simulink model "SWC_DDM_type"  (R2021b)
settings: Solver=FixedStepDiscrete  StartTime=0.0  StopTime=10.0  FixedStep=0.01  RelTol=1e-3
undefined symbols (not defined in the file): C_TASK_5MS_S, FALSE, TRUE
libraries: ddm x1
settings Model: DataDictionary=APPTypes.sldd  Creator=FVT23010  LastModifiedBy=FVT23010
settings DataIOCC: SaveFormat=StructureWithTime
settings OptimizationCC: DefaultParameterBehavior=Inlined  EnhancedBackFolding=on  PassReuseOutputArgsAs=Individual arguments  ZeroExternalMemoryAtStartup=off  ZeroInternalMemoryAtStartup=off  OptimizeBlockOrder=speed  DifferentSizesBufferReuse=on  OptimizationCustomize=off  EfficientTunableParamExpr=on
settings DebuggingCC: ParameterTunabilityLossMsg=error
settings HardwareCC: ProdBitPerPointer=32  ProdBitPerSizeT=32  ProdBitPerPtrDiffT=32  ProdLargestAtomicInteger=Long  ProdLargestAtomicFloat=Double  ProdWordSize=32  ProdLongLongMode=on  ProdHWDeviceType=ARM Compatible->ARM Cortex-M
settings ModelReferenceCC: ModelReferenceNumInstancesAllowed=Single
settings SFSimCC: MATLABDynamicMemAlloc=off
settings RTWCC: Description=AUTOSAR  SystemTargetFile=autosar.tlc  GenCodeOnly=on  TemplateMakefile=ert_default_tmf  PortableWordSizes=on
settings CodeAppCC: ForceParamTrailComments=on  IgnoreCustomStorageClasses=off  OperatorAnnotations=on  SimulinkDataObjDesc=on  SFDataObjDesc=on  InsertBlockDesc=on
settings STFCustomTargetCC: TargetLangStandard=C99 (ISO)  UtilityFuncGeneration=Shared location  MultiwordLength=256  ParMdlRefBuildCompliant=on  CompOptLevelCompliant=on  IncludeMdlTerminateFcn=off  CombineOutputUpdateFcns=on  SuppressErrorStatus=on  ERTCustomFileBanners=on  SupportNonFinite=off  SupportComplex=off  SupportContinuousTime=off  SupportNonInlinedSFcns=off  RemoveResetFunc=on  MATLABClassNameForMDSCustomization=Simulink.SoftwareTarget.ERTCustomization  AutosarCompliant=on  GRTInterface=off  UseToolchainInfoCompliant=on  GenerateSharedConstants=off  LookupTableObjectStructAxisOrder=2,1,3,4,...  LUTObjectStructOrderEvenSpacing=Size,Table,Breakpoints  SystemTargetFile=autosar.tlc
settings ERTTargetCC: TargetLangStandard=C99 (ISO)  UtilityFuncGeneration=Shared location  ConcurrentExecutionCompliant=off  IncludeMdlTerminateFcn=off  SuppressErrorStatus=on  SupportNonFinite=off  SupportComplex=off  ModelStepFunctionPrototypeControlCompliant=off  CPPClassGenCompliant=off  AutosarCompliant=on  GenerateSharedConstants=off  LookupTableObjectStructAxisOrder=2,1,3,4,...  LUTObjectStructOrderEvenSpacing=Size,Table,Breakpoints  GenerateASAP2=on  InlinedParameterPlacement=NonHierarchical  ERTCustomFileTemplate=example_file_process.tlc  ConvertIfToSwitch=off  SuppressUnreachableDefaultCases=off  BooleanTrueId=true_MatlabRTW  BooleanFalseId=false_MatlabRTW

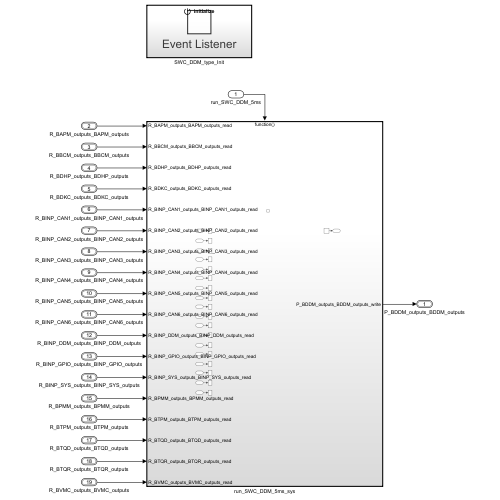
[thumbnail: Simulink's stored preview of the top-level diagram]
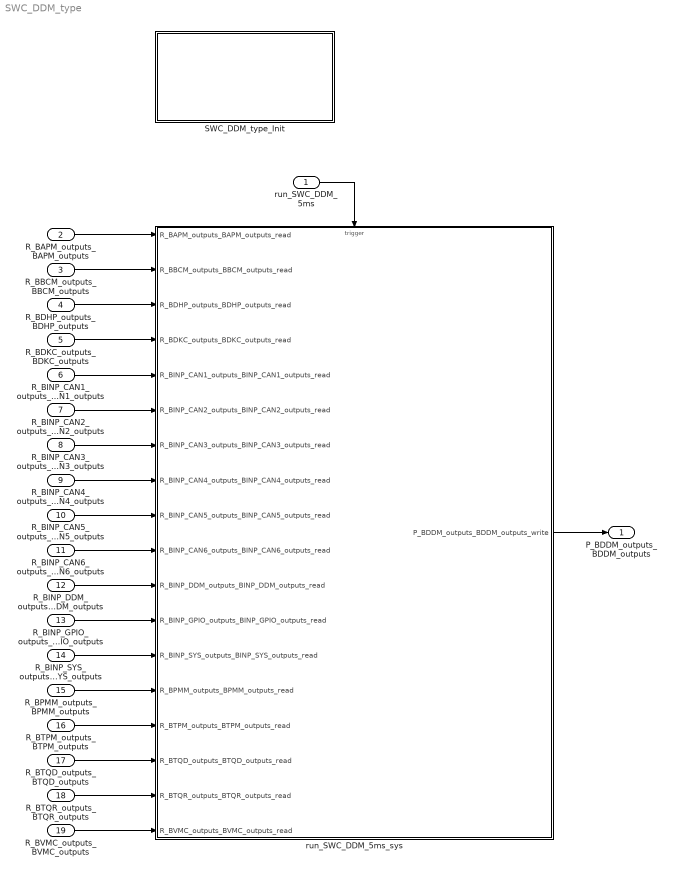
== system SWC_DDM_type ==
  run_SWC_DDM_5ms : Inport  SampleTime=0.01  OutputFunctionCall=on
  R_BAPM_outputs_BAPM_outputs : Inport  Port=2  OutDataTypeStr=Bus: BAPM_outputs  PortDimensions=1  BusOutputAsStruct=on
  R_BBCM_outputs_BBCM_outputs : Inport  Port=3  OutDataTypeStr=Bus: BBCM_outputs  PortDimensions=1  BusOutputAsStruct=on
  R_BDHP_outputs_BDHP_outputs : Inport  Port=4  OutDataTypeStr=Bus: BDHP_outputs  PortDimensions=1  BusOutputAsStruct=on
  R_BDKC_outputs_BDKC_outputs : Inport  Port=5  OutDataTypeStr=Bus: BDKC_outputs  PortDimensions=1  BusOutputAsStruct=on
  R_BINP_CAN1_outputs_BINP_CAN1_outputs : Inport  Port=6  OutDataTypeStr=Bus: BINP_CAN1_outputs  PortDimensions=1  BusOutputAsStruct=on
  R_BINP_CAN2_outputs_BINP_CAN2_outputs : Inport  Port=7  OutDataTypeStr=Bus: BINP_CAN2_outputs  PortDimensions=1  BusOutputAsStruct=on
  R_BINP_CAN3_outputs_BINP_CAN3_outputs : Inport  Port=8  OutDataTypeStr=Bus: BINP_CAN3_outputs  PortDimensions=1  BusOutputAsStruct=on
  R_BINP_CAN4_outputs_BINP_CAN4_outputs : Inport  Port=9  OutDataTypeStr=Bus: BINP_CAN4_outputs  PortDimensions=1  BusOutputAsStruct=on
  R_BINP_CAN5_outputs_BINP_CAN5_outputs : Inport  Port=10  OutDataTypeStr=Bus: BINP_CAN5_outputs  PortDimensions=1  BusOutputAsStruct=on
  R_BINP_CAN6_outputs_BINP_CAN6_outputs : Inport  Port=11  OutDataTypeStr=Bus: BINP_CAN6_outputs  PortDimensions=1  BusOutputAsStruct=on
  R_BINP_DDM_outputs_BINP_DDM_outputs : Inport  Port=12  OutDataTypeStr=Bus: BINP_DDM_outputs  PortDimensions=1  BusOutputAsStruct=on
  R_BINP_GPIO_outputs_BINP_GPIO_outputs : Inport  Port=13  OutDataTypeStr=Bus: BINP_GPIO_outputs  PortDimensions=1  BusOutputAsStruct=on
  R_BINP_SYS_outputs_BINP_SYS_outputs : Inport  Port=14  OutDataTypeStr=Bus: BINP_SYS_outputs  PortDimensions=1  BusOutputAsStruct=on
  R_BPMM_outputs_BPMM_outputs : Inport  Port=15  OutDataTypeStr=Bus: BPMM_outputs  PortDimensions=1  BusOutputAsStruct=on
  R_BTPM_outputs_BTPM_outputs : Inport  Port=16  OutDataTypeStr=Bus: BTPM_outputs  PortDimensions=1  BusOutputAsStruct=on
  R_BTQD_outputs_BTQD_outputs : Inport  Port=17  OutDataTypeStr=Bus: BTQD_outputs  PortDimensions=1  BusOutputAsStruct=on
  R_BTQR_outputs_BTQR_outputs : Inport  Port=18  OutDataTypeStr=Bus: BTQR_outputs  PortDimensions=1  BusOutputAsStruct=on
  R_BVMC_outputs_BVMC_outputs : Inport  Port=19  OutDataTypeStr=Bus: BVMC_outputs  PortDimensions=1  BusOutputAsStruct=on
  SWC_DDM_type_Init : Subsystem
  run_SWC_DDM_5ms_sys : Subsystem
  P_BDDM_outputs_BDDM_outputs : Outport  OutDataTypeStr=Bus: BDDM_outputs  PortDimensions=1  BusOutputAsStruct=on
  wires:
  R_BAPM_outputs_BAPM_outputs/1 -> run_SWC_DDM_5ms_sys/1(R_BAPM_outputs_BAPM_outputs_read)
  R_BBCM_outputs_BBCM_outputs/1 -> run_SWC_DDM_5ms_sys/2(R_BBCM_outputs_BBCM_outputs_read)
  R_BDHP_outputs_BDHP_outputs/1 -> run_SWC_DDM_5ms_sys/3(R_BDHP_outputs_BDHP_outputs_read)
  R_BDKC_outputs_BDKC_outputs/1 -> run_SWC_DDM_5ms_sys/4(R_BDKC_outputs_BDKC_outputs_read)
  R_BINP_CAN1_outputs_BINP_CAN1_outputs/1 -> run_SWC_DDM_5ms_sys/5(R_BINP_CAN1_outputs_BINP_CAN1_outputs_read)
  R_BINP_CAN2_outputs_BINP_CAN2_outputs/1 -> run_SWC_DDM_5ms_sys/6(R_BINP_CAN2_outputs_BINP_CAN2_outputs_read)
  R_BINP_CAN3_outputs_BINP_CAN3_outputs/1 -> run_SWC_DDM_5ms_sys/7(R_BINP_CAN3_outputs_BINP_CAN3_outputs_read)
  R_BINP_CAN4_outputs_BINP_CAN4_outputs/1 -> run_SWC_DDM_5ms_sys/8(R_BINP_CAN4_outputs_BINP_CAN4_outputs_read)
  R_BINP_CAN5_outputs_BINP_CAN5_outputs/1 -> run_SWC_DDM_5ms_sys/9(R_BINP_CAN5_outputs_BINP_CAN5_outputs_read)
  R_BINP_CAN6_outputs_BINP_CAN6_outputs/1 -> run_SWC_DDM_5ms_sys/10(R_BINP_CAN6_outputs_BINP_CAN6_outputs_read)
  R_BINP_DDM_outputs_BINP_DDM_outputs/1 -> run_SWC_DDM_5ms_sys/11(R_BINP_DDM_outputs_BINP_DDM_outputs_read)
  R_BINP_GPIO_outputs_BINP_GPIO_outputs/1 -> run_SWC_DDM_5ms_sys/12(R_BINP_GPIO_outputs_BINP_GPIO_outputs_read)
  R_BINP_SYS_outputs_BINP_SYS_outputs/1 -> run_SWC_DDM_5ms_sys/13(R_BINP_SYS_outputs_BINP_SYS_outputs_read)
  R_BPMM_outputs_BPMM_outputs/1 -> run_SWC_DDM_5ms_sys/14(R_BPMM_outputs_BPMM_outputs_read)
  R_BTPM_outputs_BTPM_outputs/1 -> run_SWC_DDM_5ms_sys/15(R_BTPM_outputs_BTPM_outputs_read)
  R_BTQD_outputs_BTQD_outputs/1 -> run_SWC_DDM_5ms_sys/16(R_BTQD_outputs_BTQD_outputs_read)
  R_BTQR_outputs_BTQR_outputs/1 -> run_SWC_DDM_5ms_sys/17(R_BTQR_outputs_BTQR_outputs_read)
  R_BVMC_outputs_BVMC_outputs/1 -> run_SWC_DDM_5ms_sys/18(R_BVMC_outputs_BVMC_outputs_read)
  run_SWC_DDM_5ms_sys/1(P_BDDM_outputs_BDDM_outputs_write) -> P_BDDM_outputs_BDDM_outputs/1
  run_SWC_DDM_5ms/1 -> run_SWC_DDM_5ms_sys/Trigger

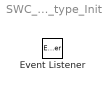
== system SWC_DDM_type/SWC_DDM_type_Init ==
  Event Listener : EventListener  EventName=reset

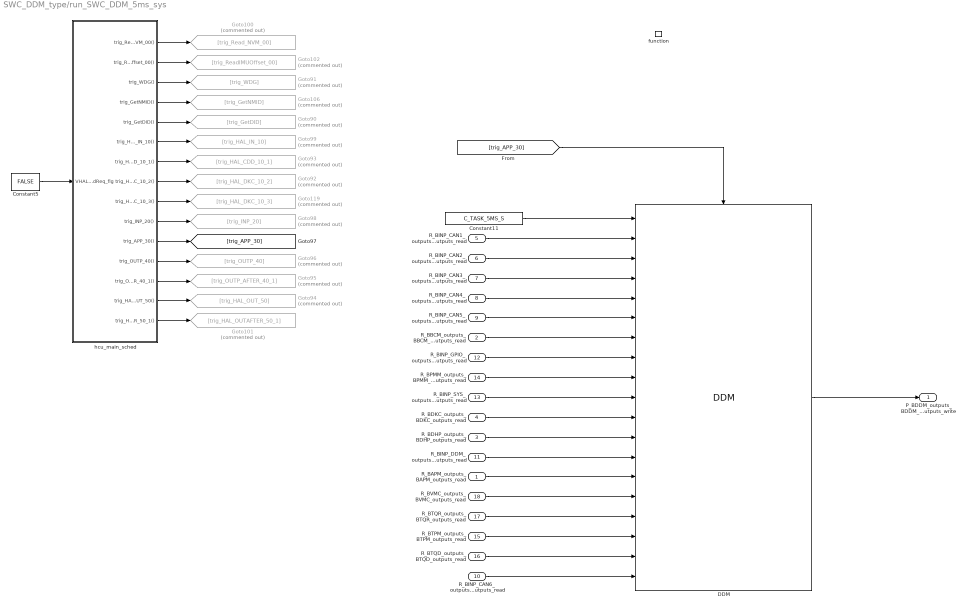
== system SWC_DDM_type/run_SWC_DDM_5ms_sys ==
  R_BAPM_outputs_BAPM_outputs_read : Inport
  R_BBCM_outputs_BBCM_outputs_read : Inport  Port=2
  R_BDHP_outputs_BDHP_outputs_read : Inport  Port=3
  R_BDKC_outputs_BDKC_outputs_read : Inport  Port=4
  R_BINP_CAN1_outputs_BINP_CAN1_outputs_read : Inport  Port=5
  R_BINP_CAN2_outputs_BINP_CAN2_outputs_read : Inport  Port=6
  R_BINP_CAN3_outputs_BINP_CAN3_outputs_read : Inport  Port=7
  R_BINP_CAN4_outputs_BINP_CAN4_outputs_read : Inport  Port=8
  R_BINP_CAN5_outputs_BINP_CAN5_outputs_read : Inport  Port=9
  R_BINP_CAN6_outputs_BINP_CAN6_outputs_read : Inport  Port=10
  R_BINP_DDM_outputs_BINP_DDM_outputs_read : Inport  Port=11
  R_BINP_GPIO_outputs_BINP_GPIO_outputs_read : Inport  Port=12
  R_BINP_SYS_outputs_BINP_SYS_outputs_read : Inport  Port=13
  R_BPMM_outputs_BPMM_outputs_read : Inport  Port=14
  R_BTPM_outputs_BTPM_outputs_read : Inport  Port=15
  R_BTQD_outputs_BTQD_outputs_read : Inport  Port=16
  R_BTQR_outputs_BTQR_outputs_read : Inport  Port=17
  R_BVMC_outputs_BVMC_outputs_read : Inport  Port=18
  function : TriggerPort  TriggerType=function-call  VariantControl=(inherit)  SampleTimeType=periodic  SampleTime=-1
  Constant11 : Constant  Value=C_TASK_5MS_S  OutDataTypeStr=single
  Constant5 : Constant  Value=FALSE
  DDM : ddm/DDM  SystemSampleTime=-1  VariantActivationTime=update diagram  Latency=0  AutoFrameSizeCalculation=off
  Goto100 : Goto  Commented=on  GotoTag=trig_Read_NVM_00
  Goto101 : Goto  Commented=on  GotoTag=trig_HAL_OUTAFTER_50_1
  Goto102 : Goto  Commented=on  GotoTag=trig_ReadIMUOffset_00
  Goto106 : Goto  Commented=on  GotoTag=trig_GetNMID
  Goto119 : Goto  Commented=on  GotoTag=trig_HAL_DKC_10_3
  Goto90 : Goto  Commented=on  GotoTag=trig_GetDID
  Goto91 : Goto  Commented=on  GotoTag=trig_WDG
  Goto92 : Goto  Commented=on  GotoTag=trig_HAL_DKC_10_2
  Goto93 : Goto  Commented=on  GotoTag=trig_HAL_CDD_10_1
  Goto94 : Goto  Commented=on  GotoTag=trig_HAL_OUT_50
  Goto95 : Goto  Commented=on  GotoTag=trig_OUTP_AFTER_40_1
  Goto96 : Goto  Commented=on  GotoTag=trig_OUTP_40
  Goto98 : Goto  Commented=on  GotoTag=trig_INP_20
  Goto99 : Goto  Commented=on  GotoTag=trig_HAL_IN_10
  hcu_main_sched : Stateflow chart  TreatAsAtomicUnit=on
  P_BDDM_outputs_BDDM_outputs_write : Outport
  wires:
  Constant11/1 -> DDM/1
  R_BINP_CAN1_outputs_BINP_CAN1_outputs_read/1 -> DDM/2
  R_BINP_CAN2_outputs_BINP_CAN2_outputs_read/1 -> DDM/3
  R_BINP_CAN3_outputs_BINP_CAN3_outputs_read/1 -> DDM/4
  R_BINP_CAN4_outputs_BINP_CAN4_outputs_read/1 -> DDM/5
  R_BINP_CAN5_outputs_BINP_CAN5_outputs_read/1 -> DDM/6
  R_BBCM_outputs_BBCM_outputs_read/1 -> DDM/7
  R_BINP_GPIO_outputs_BINP_GPIO_outputs_read/1 -> DDM/8
  R_BPMM_outputs_BPMM_outputs_read/1 -> DDM/9
  R_BINP_SYS_outputs_BINP_SYS_outputs_read/1 -> DDM/10
  R_BDKC_outputs_BDKC_outputs_read/1 -> DDM/11
  R_BDHP_outputs_BDHP_outputs_read/1 -> DDM/12
  R_BINP_DDM_outputs_BINP_DDM_outputs_read/1 -> DDM/13
  R_BAPM_outputs_BAPM_outputs_read/1 -> DDM/14
  R_BVMC_outputs_BVMC_outputs_read/1 -> DDM/15
  R_BTQR_outputs_BTQR_outputs_read/1 -> DDM/16
  R_BTPM_outputs_BTPM_outputs_read/1 -> DDM/17
  R_BTQD_outputs_BTQD_outputs_read/1 -> DDM/18
  R_BINP_CAN6_outputs_BINP_CAN6_outputs_read/1 -> DDM/19
  DDM/1 -> P_BDDM_outputs_BDDM_outputs_write/1
  hcu_main_sched/10(trig_INP_20()) -> Goto98/1
  hcu_main_sched/12(trig_OUTP_40()) -> Goto96/1
  hcu_main_sched/14(trig_HAL_OUT_50()) -> Goto94/1
  hcu_main_sched/2(trig_ReadIMUOffset_00()) -> Goto102/1
  hcu_main_sched/15(trig_HAL_OUTAFTER_50_1()) -> Goto101/1
  hcu_main_sched/1(trig_Read_NVM_00()) -> Goto100/1
  hcu_main_sched/11(trig_APP_30()) -> [trig_APP_30]
  hcu_main_sched/5(trig_GetDID()) -> Goto90/1
  hcu_main_sched/4(trig_GetNMID()) -> Goto106/1
  Constant5/1 -> hcu_main_sched/1(VHAL_FusionSchedReq_flg)
  hcu_main_sched/9(trig_HAL_DKC_10_3()) -> Goto119/1
  hcu_main_sched/6(trig_HAL_IN_10()) -> Goto99/1
  hcu_main_sched/8(trig_HAL_DKC_10_2()) -> Goto92/1
  hcu_main_sched/3(trig_WDG()) -> Goto91/1
  hcu_main_sched/7(trig_HAL_CDD_10_1()) -> Goto93/1
  hcu_main_sched/13(trig_OUTP_AFTER_40_1()) -> Goto95/1
  [trig_APP_30] -> DDM/Trigger

== stateflow chart SWC_DDM_type/run_SWC_DDM_5ms_sys/hcu_main_sched ==
  state Main_Scheduler
    (default) -> (junction 31) : {
        |   Sys_Init_done = FALSE;
        |   trig_Read_NVM_00;
        |   trig_ReadIMUOffset_00;
        | }
    Main_Scheduler -> (junction 31) : {Sys_Init_done = TRUE;}
    (junction 31) -> (junction 34) [order 1] : [
        |    Sys_Init_done &&...
        |    !VHAL_FusionSchedReq_flg
        | ]
    (junction 31) -> (junction 38) [order 2]
    (junction 34) -> (junction 36) : {
        |     trig_WDG;
        |     trig_GetNMID;
        |     trig_GetDID;
        |     trig_HAL_IN_10;
        |     trig_HAL_CDD_10_1;
        |     trig_HAL_DKC_10_2;
        |     trig_HAL_DKC_10_3;
        |     trig_INP_20;
        |     trig_APP_30;
        |     trig_OUTP_40;
        |     trig_OUTP_AFTER_40_1;
        |     trig_HAL_OUT_50;
        |     trig_HAL_OUTAFTER_50_1;
        |    }
    (junction 36) -> (junction 38)
  (default) -> Main_Scheduler
  data: VHAL_FusionSchedReq_flg input; Sys_Init_done local double; FALSE parameter; TRUE parameter
  events: trig_Read_NVM_00 output FUNCTION_CALL_EVENT; trig_ReadIMUOffset_00 output FUNCTION_CALL_EVENT; trig_WDG output FUNCTION_CALL_EVENT; trig_GetNMID output FUNCTION_CALL_EVENT; trig_GetDID output FUNCTION_CALL_EVENT; trig_HAL_IN_10 output FUNCTION_CALL_EVENT; trig_HAL_CDD_10_1 output FUNCTION_CALL_EVENT; trig_HAL_DKC_10_2 output FUNCTION_CALL_EVENT; trig_HAL_DKC_10_3 output FUNCTION_CALL_EVENT; trig_INP_20 output FUNCTION_CALL_EVENT; trig_APP_30 output FUNCTION_CALL_EVENT; trig_OUTP_40 output FUNCTION_CALL_EVENT; trig_OUTP_AFTER_40_1 output FUNCTION_CALL_EVENT; trig_HAL_OUT_50 output FUNCTION_CALL_EVENT; trig_HAL_OUTAFTER_50_1 output FUNCTION_CALL_EVENT
